simulink model "omav_LBF_hover"  (R2020a)
settings: Solver=VariableStepAuto  StartTime=0.0  StopTime=20  RelTol=1e-3
undefined symbols (not defined in the file): params
libraries: simulink x12, vrlib x1
settings Model: Creator=daniel  LastModifiedBy=daniel

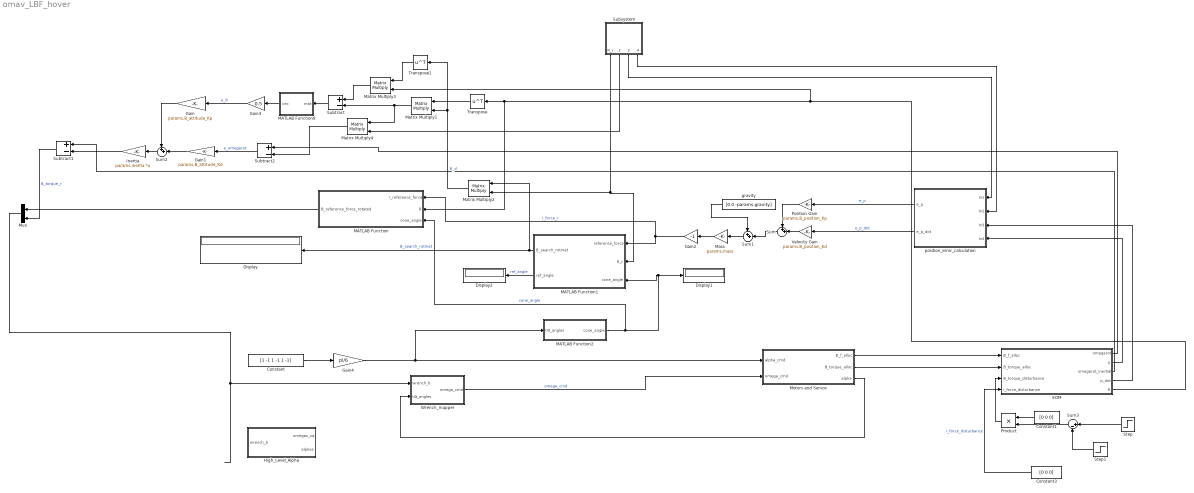
== system omav_LBF_hover ==
  Constant : Constant  Value=[1 -1 1 -1 1 -1]
  Constant1 : Constant  Value=[0 0 0]
  Constant3 : Constant  Value=[0 0 0]
  Display : Display
  Display1 : Display
  Display2 : Display
  EOM : Subsystem
  Gain : Gain  Gain=params.B_attitude_Kp
  Gain1 : Gain  Gain=params.B_attitude_Kd
  Gain2 : Gain  Gain=-1
  Gain3 : Gain  Gain=0.5
  Gain4 : Gain  Gain=pi/6
  High_Level_Alpha : Subsystem
  Inertia : Gain  Gain=params.inertia  Multiplication=Matrix(K*u) (u vector)
  MATLAB Function : MATLAB Function  TreatAsAtomicUnit=on
  MATLAB Function1 : MATLAB Function  TreatAsAtomicUnit=on
  MATLAB Function2 : MATLAB Function  TreatAsAtomicUnit=on
  MATLAB Function8 : MATLAB Function  TreatAsAtomicUnit=on
  Mass : Gain  Gain=params.mass
  Matrix Multiply{1..4} (4 alike) : Product  Multiplication=Matrix(*)
  Motors and Servos : Subsystem
  Mux : Mux  Inputs=2
  Position Gain : Gain  Gain=params.B_position_Kp
  Product : Product
  Step : Step  SampleTime=0
  Step1 : Step  Time=3  SampleTime=0
  Subsystem : Subsystem
  Subtract : Sum  Inputs=+-
  Subtract1 : Sum  Inputs=+-
  Subtract2 : Sum  Inputs=+-
  Sum : Sum  Inputs=++|
  Sum1 : Sum  Inputs=++|
  Sum2 : Sum  Inputs=++|
  Sum3 : Sum  Inputs=|+-
  Transpose : Math  Operator=transpose  SaturateOnIntegerOverflow=on
  Transpose1 : Math  Operator=transpose  SaturateOnIntegerOverflow=on
  Velocity Gain : Gain  Gain=params.B_position_Kd
  Wrench_mapper : Subsystem
  gravity : Constant  Value=[0 0 -params.gravity]
  position_error_calculation : Subsystem
  wires:
  Mux/1 -> Wrench_mapper/1(wrench_b)
  Constant3/1 -> EOM/4(I_force_disturbance)  "I_force_disturbance"
  Motors and Servos/1(B_f_alloc) -> EOM/1(B_f_alloc)
  Motors and Servos/2(B_torque_alloc) -> EOM/2(B_torque_alloc)
  Constant/1 -> Gain4/1
  Motors and Servos/3(alpha) -> Wrench_mapper/2(tilt_angles)
  Wrench_mapper/1(omega_cmd) -> Motors and Servos/2(omega_cmd)  "omega_cmd"
  Velocity Gain/1 -> Sum/2
  Position Gain/1 -> Sum/1
  Sum/1 -> Sum1/2
  gravity/1 -> Sum1/1
  Sum1/1 -> Mass/1
  Gain2/1 -> MATLAB Function1/1(reference_force), MATLAB Function/1(I_reference_force)  "I_force_r"
  MATLAB Function1/1(B_search_rotmat) -> Display/1, Matrix Multiply2/1  "B_search_rotmat"
  Matrix Multiply1/1 -> Subtract/2, Matrix Multiply4/1
  Matrix Multiply4/1 -> Subtract2/2
  EOM/4(p_dot) -> position_error_calculation/3(In3)
  Matrix Multiply3/1 -> Subtract/1
  EOM/5(R) -> Matrix Multiply3/2, MATLAB Function/2(R), Transpose/1
  Transpose1/1 -> Matrix Multiply3/1
  MATLAB Function8/1(vec) -> Gain3/1
  Subtract2/1 -> Gain1/1  "e_omegarot"
  Subtract/1 -> MATLAB Function8/1(mat)
  Transpose/1 -> Matrix Multiply1/1
  EOM/1(omegarot) -> Subtract2/1
  Gain3/1 -> Gain/1  "e_R"
  EOM/2(p) -> position_error_calculation/4(In4)
  position_error_calculation/1(e_p) -> Position Gain/1  "e_p"
  position_error_calculation/2(e_p_dot) -> Velocity Gain/1  "e_p_dot"
  Matrix Multiply2/1 -> Matrix Multiply1/2, Transpose1/1  "R_d"
  Subsystem/2(omega_dot_r) -> Matrix Multiply4/2
  Subsystem/3(Out3) -> position_error_calculation/1(In1)
  Subsystem/4(p_r1) -> position_error_calculation/2(In2)
  Subsystem/1(R_r) -> MATLAB Function1/2(R_r), Matrix Multiply2/2
  EOM/3(omegarot_inertial) -> Subtract1/1
  Gain1/1 -> Sum2/2
  Gain/1 -> Sum2/1
  Sum2/1 -> Inertia/1
  Inertia/1 -> Subtract1/2
  Subtract1/1 -> Mux/2  "B_torque_r"
  Mass/1 -> Gain2/1
  Step/1 -> Sum3/1
  Step1/1 -> Sum3/2
  Sum3/1 -> Product/2
  Constant1/1 -> Product/1
  Product/1 -> EOM/3(B_torque_disturbance)
  Gain4/1 -> MATLAB Function2/1(tilt_angles), Motors and Servos/1(alpha_cmd)
  MATLAB Function2/1(cone_angle) -> MATLAB Function/3(cone_angle), Display1/1, MATLAB Function1/3(cone_angle)  "cone_angle"
  MATLAB Function/1(B_reference_force_rotated) -> Mux/1
  MATLAB Function1/2(ref_angle) -> Display2/1  "ref_angle"

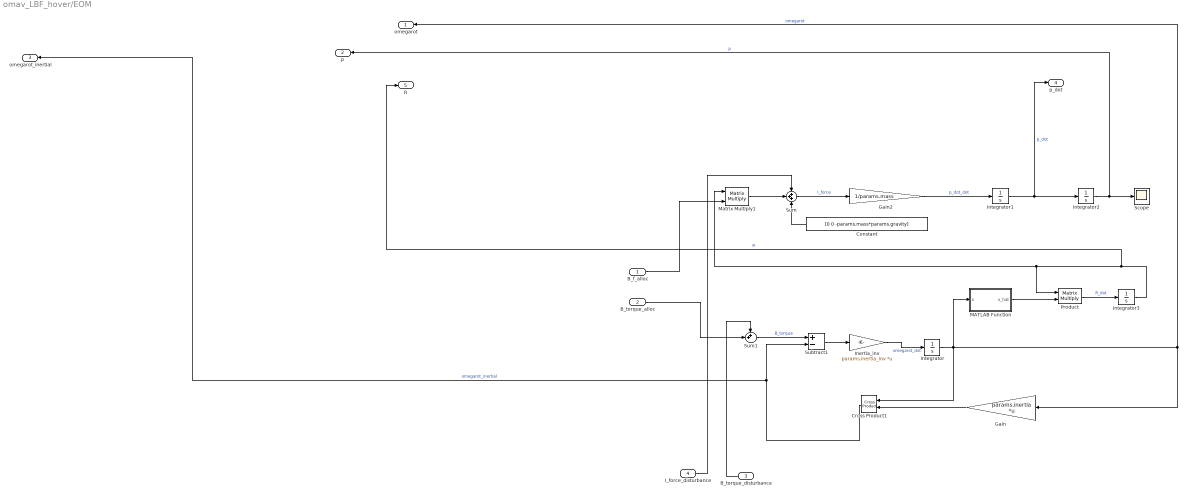
== system omav_LBF_hover/EOM ==
  B_f_alloc : Inport
  B_torque_alloc : Inport  Port=2
  B_torque_disturbance : Inport  Port=3
  I_force_disturbance : Inport  Port=4
  Constant : Constant  Value=[0 0 -params.mass*params.gravity]
  Cross Product1 : vrlib/Utilities/Cross Product
  Gain : Gain  Gain=params.inertia  Multiplication=Matrix(K*u) (u vector)
  Gain2 : Gain  Gain=1/params.mass
  Inertia_inv : Gain  Gain=params.inertia_inv  Multiplication=Matrix(K*u) (u vector)
  Integrator : Integrator
  Integrator1 : Integrator
  Integrator2 : Integrator
  Integrator3 : Integrator  InitialCondition=[1 0 0;0 1 0;0 0 1]
  MATLAB Function : MATLAB Function  TreatAsAtomicUnit=on
  Matrix Multiply1 : Product  Multiplication=Matrix(*)
  Product : Product  Multiplication=Matrix(*)  OutMin=0
  Scope : Scope
  Subtract1 : Sum  Inputs=+-
  Sum : Sum  Inputs=+++
  Sum1 : Sum  Inputs=++|
  omegarot : Outport
  p : Outport  Port=2
  omegarot_inertial : Outport  Port=3
  p_dot : Outport  Port=4
  R : Outport  Port=5
  wires:
  MATLAB Function/1(x_hat) -> Product/2
  Inertia_inv/1 -> Integrator/1  "omegarot_dot"
  Matrix Multiply1/1 -> Sum/2
  Sum1/1 -> Subtract1/1  "B_torque"
  Sum/1 -> Gain2/1  "I_force"
  B_torque_disturbance/1 -> Sum1/1
  Constant/1 -> Sum/3
  Integrator3/1 -> R/1, Product/1, Matrix Multiply1/1  "R"
  Integrator2/1 -> p/1, Scope/1  "p"
  Gain/1 -> Cross Product1/2
  Product/1 -> Integrator3/1  "R_dot"
  Subtract1/1 -> Inertia_inv/1
  Gain2/1 -> Integrator1/1  "p_dot_dot"
  B_f_alloc/1 -> Matrix Multiply1/2
  Cross Product1/1 -> omegarot_inertial/1, Subtract1/2  "omegarot_inertial"
  B_torque_alloc/1 -> Sum1/2
  Integrator/1 -> omegarot/1, Gain/1, MATLAB Function/1(x), Cross Product1/1  "omegarot"
  I_force_disturbance/1 -> Sum/1
  Integrator1/1 -> p_dot/1, Integrator2/1  "p_dot"

== system omav_LBF_hover/High_Level_Alpha ==
  wrench_b : Inport
  MATLAB Function3 : MATLAB Function  TreatAsAtomicUnit=on
  MATLAB Function4 : MATLAB Function  TreatAsAtomicUnit=on
  MATLAB Function5 : MATLAB Function  TreatAsAtomicUnit=on
  omegas_sq : Outport
  alphas : Outport  Port=2
  wires:
  MATLAB Function5/1(X) -> MATLAB Function4/1(X)
  wrench_b/1 -> MATLAB Function5/2(wrench_b)
  MATLAB Function4/2(omegas_sq) -> omegas_sq/1
  MATLAB Function4/1(alphas) -> alphas/1
  MATLAB Function3/1(A) -> MATLAB Function5/1(A)

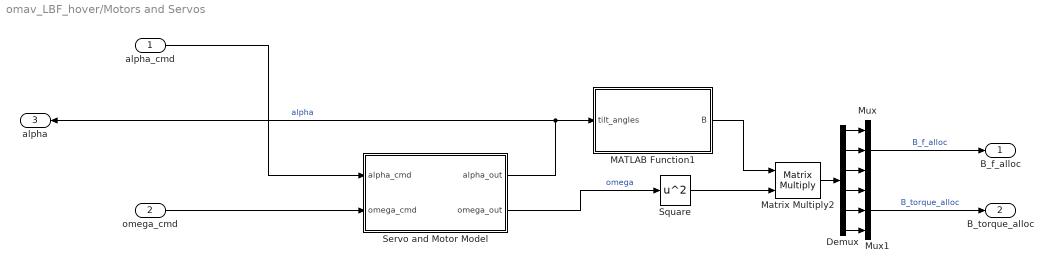
== system omav_LBF_hover/Motors and Servos ==
  alpha_cmd : Inport
  omega_cmd : Inport  Port=2
  Demux : Demux  Outputs=6
  MATLAB Function1 : MATLAB Function  TreatAsAtomicUnit=on
  Matrix Multiply2 : Product  Multiplication=Matrix(*)
  Mux : Mux  Inputs=3
  Mux1 : Mux  Inputs=3
  Servo and Motor Model : Subsystem
  Square : Math  Operator=square  SaturateOnIntegerOverflow=on
  B_f_alloc : Outport
  B_torque_alloc : Outport  Port=2
  alpha : Outport  Port=3
  wires:
  Demux/1 -> Mux/1
  MATLAB Function1/1(B) -> Matrix Multiply2/1
  Demux/4 -> Mux1/1
  Servo and Motor Model/2(omega_out) -> Square/1  "omega"
  Demux/5 -> Mux1/2
  Matrix Multiply2/1 -> Demux/1
  Servo and Motor Model/1(alpha_out) -> alpha/1, MATLAB Function1/1(tilt_angles)  "alpha"
  alpha_cmd/1 -> Servo and Motor Model/1(alpha_cmd)
  Demux/6 -> Mux1/3
  Demux/2 -> Mux/2
  Square/1 -> Matrix Multiply2/2
  omega_cmd/1 -> Servo and Motor Model/2(omega_cmd)
  Mux/1 -> B_f_alloc/1  "B_f_alloc"
  Demux/3 -> Mux/3
  Mux1/1 -> B_torque_alloc/1  "B_torque_alloc"

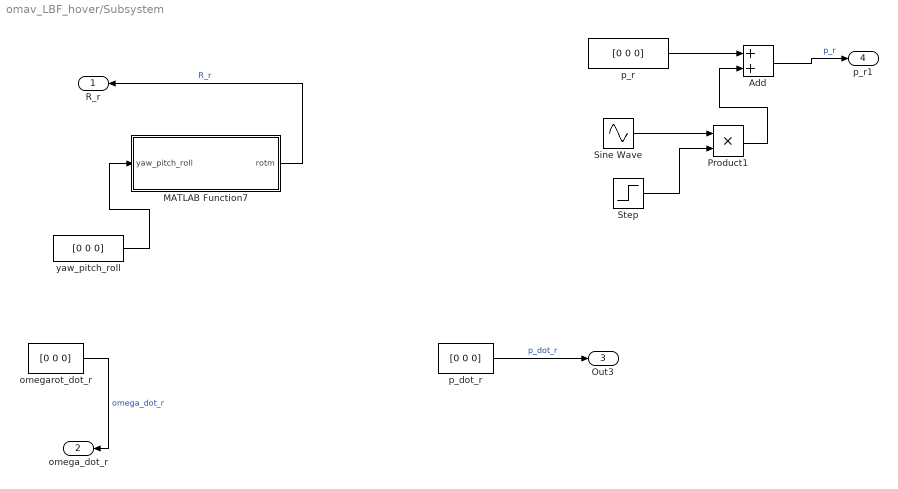
== system omav_LBF_hover/Subsystem ==
  Add : Sum
  MATLAB Function7 : MATLAB Function  TreatAsAtomicUnit=on
  Product1 : Product
  Sine Wave : Sin  Amplitude=[1 0 0]  Frequency=2  SampleTime=0
  Step : Step  Time=3  SampleTime=0
  omegarot_dot_r : Constant  Value=[0 0 0]
  p_dot_r : Constant  Value=[0 0 0]
  p_r : Constant  Value=[0 0 0]
  yaw_pitch_roll : Constant  Value=[0 0 0]
  R_r : Outport
  omega_dot_r : Outport  Port=2
  Out3 : Outport  Port=3
  p_r1 : Outport  Port=4
  wires:
  Step/1 -> Product1/2
  omegarot_dot_r/1 -> omega_dot_r/1  "omega_dot_r"
  Add/1 -> p_r1/1  "p_r"
  yaw_pitch_roll/1 -> MATLAB Function7/1(yaw_pitch_roll)
  MATLAB Function7/1(rotm) -> R_r/1  "R_r"
  Product1/1 -> Add/2
  p_dot_r/1 -> Out3/1  "p_dot_r"
  Sine Wave/1 -> Product1/1
  p_r/1 -> Add/1

== system omav_LBF_hover/Wrench_mapper ==
  wrench_b : Inport
  tilt_angles : Inport  Port=2
  MATLAB Function2 : MATLAB Function  TreatAsAtomicUnit=on
  MATLAB Function6 : MATLAB Function  TreatAsAtomicUnit=on
  Sqrt : Sqrt  SaturateOnIntegerOverflow=on
  omega_cmd : Outport
  wires:
  wrench_b/1 -> MATLAB Function2/2(wrench_b)
  Sqrt/1 -> omega_cmd/1  "omega_cmd"
  MATLAB Function2/1(omega_sq) -> Sqrt/1
  MATLAB Function6/1(B) -> MATLAB Function2/1(B)
  tilt_angles/1 -> MATLAB Function6/1(tilt_angles)

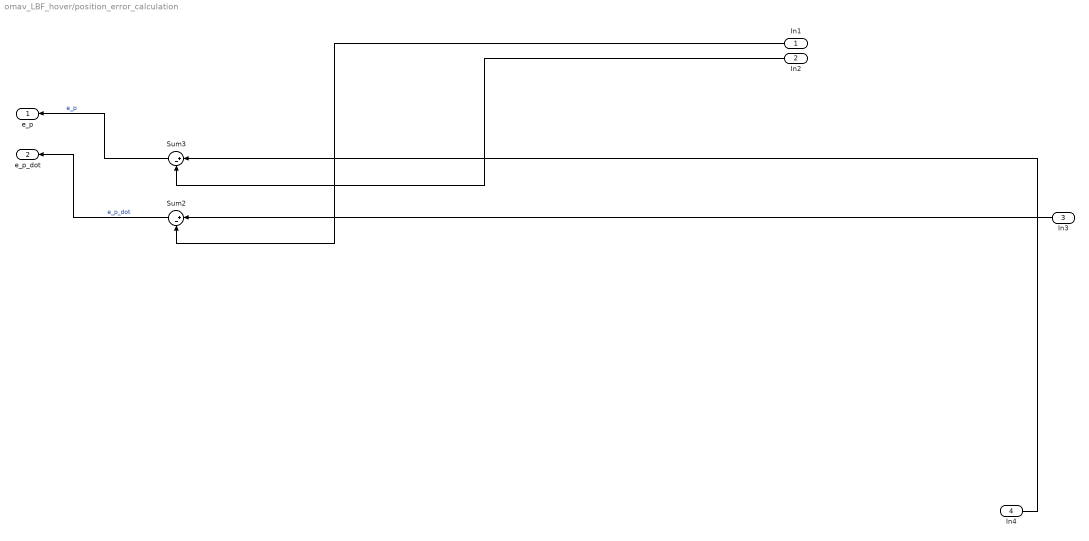
== system omav_LBF_hover/position_error_calculation ==
  In1 : Inport
  In2 : Inport  Port=2
  In3 : Inport  Port=3
  In4 : Inport  Port=4
  Sum2 : Sum  Inputs=|+-
  Sum3 : Sum  Inputs=|+-
  e_p : Outport
  e_p_dot : Outport  Port=2
  wires:
  Sum2/1 -> e_p_dot/1  "e_p_dot"
  In3/1 -> Sum2/1
  In4/1 -> Sum3/1
  In1/1 -> Sum2/2
  Sum3/1 -> e_p/1  "e_p"
  In2/1 -> Sum3/2

== system omav_LBF_hover/Motors and Servos/Servo and Motor Model ==
  alpha_cmd : Inport
  omega_cmd : Inport  Port=2
  all_rotors_subsystem1 : Subsystem
      mask Display: image('images/brushless.JPG'); % Use "Edit Image" on toolstrip to change.
  all_servos_subsystem1 : Subsystem
      mask Display: image('images/servo.jpg'); % Use "Edit Image" on toolstrip to change.
  alpha_out : Outport
  omega_out : Outport  Port=2
  wires:
  alpha_cmd/1 -> all_servos_subsystem1/1(alphas_cmd)  "alpha_cmd"
  all_rotors_subsystem1/1(omegas_out) -> omega_out/1  "omega_out"
  all_servos_subsystem1/1(alphas_out) -> alpha_out/1  "alpha_out"
  omega_cmd/1 -> all_rotors_subsystem1/1(omegas_cmd)  "omega_cmd"

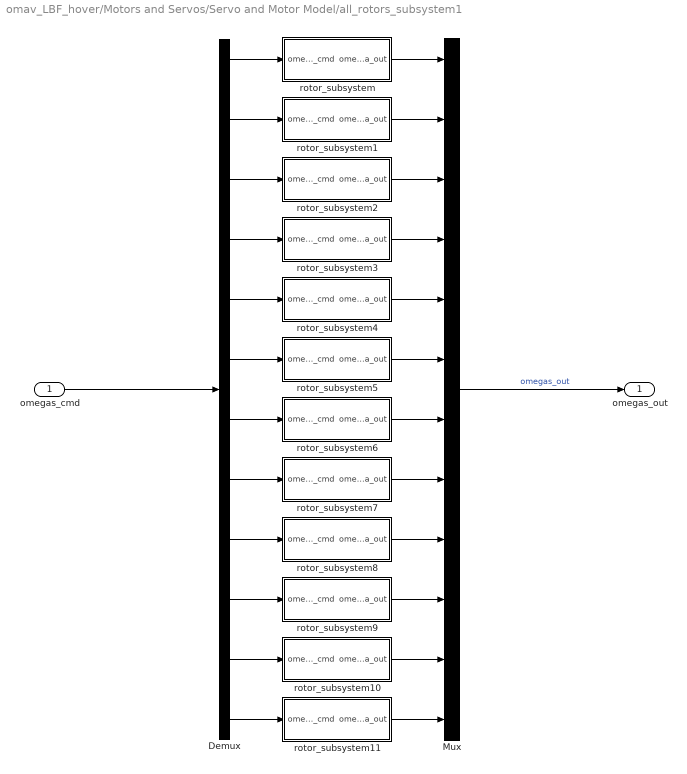
== system omav_LBF_hover/Motors and Servos/Servo and Motor Model/all_rotors_subsystem1 ==
  omegas_cmd : Inport
  Demux : Demux  Outputs=12
  Mux : Mux  Inputs=12
  rotor_subsystem : Subsystem
  rotor_subsystem1 : Subsystem
  rotor_subsystem10 : Subsystem
  rotor_subsystem11 : Subsystem
  rotor_subsystem2 : Subsystem
  rotor_subsystem3 : Subsystem
  rotor_subsystem4 : Subsystem
  rotor_subsystem5 : Subsystem
  rotor_subsystem6 : Subsystem
  rotor_subsystem7 : Subsystem
  rotor_subsystem8 : Subsystem
  rotor_subsystem9 : Subsystem
  omegas_out : Outport
  wires:
  Demux/3 -> rotor_subsystem2/1(omega_cmd)
  rotor_subsystem10/1(omega_out) -> Mux/11
  rotor_subsystem7/1(omega_out) -> Mux/8
  rotor_subsystem2/1(omega_out) -> Mux/3
  rotor_subsystem1/1(omega_out) -> Mux/2
  Demux/2 -> rotor_subsystem1/1(omega_cmd)
  rotor_subsystem5/1(omega_out) -> Mux/6
  rotor_subsystem4/1(omega_out) -> Mux/5
  Demux/4 -> rotor_subsystem3/1(omega_cmd)
  rotor_subsystem6/1(omega_out) -> Mux/7
  Demux/8 -> rotor_subsystem7/1(omega_cmd)
  rotor_subsystem/1(omega_out) -> Mux/1
  rotor_subsystem3/1(omega_out) -> Mux/4
  rotor_subsystem11/1(omega_out) -> Mux/12
  rotor_subsystem8/1(omega_out) -> Mux/9
  Demux/11 -> rotor_subsystem10/1(omega_cmd)
  rotor_subsystem9/1(omega_out) -> Mux/10
  Demux/1 -> rotor_subsystem/1(omega_cmd)
  omegas_cmd/1 -> Demux/1
  Mux/1 -> omegas_out/1  "omegas_out"
  Demux/12 -> rotor_subsystem11/1(omega_cmd)
  Demux/10 -> rotor_subsystem9/1(omega_cmd)
  Demux/9 -> rotor_subsystem8/1(omega_cmd)
  Demux/7 -> rotor_subsystem6/1(omega_cmd)
  Demux/6 -> rotor_subsystem5/1(omega_cmd)
  Demux/5 -> rotor_subsystem4/1(omega_cmd)

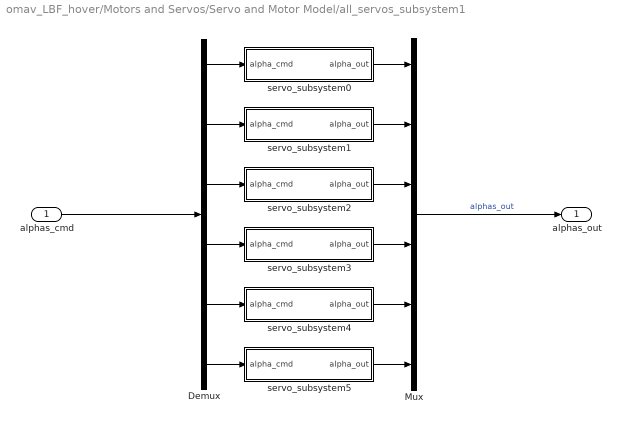
== system omav_LBF_hover/Motors and Servos/Servo and Motor Model/all_servos_subsystem1 ==
  alphas_cmd : Inport
  Demux : Demux  Outputs=6
  Mux : Mux  Inputs=6
  servo_subsystem0 : Subsystem
  servo_subsystem1 : Subsystem
  servo_subsystem2 : Subsystem
  servo_subsystem3 : Subsystem
  servo_subsystem4 : Subsystem
  servo_subsystem5 : Subsystem
  alphas_out : Outport
  wires:
  alphas_cmd/1 -> Demux/1
  Demux/2 -> servo_subsystem1/1(alpha_cmd)
  servo_subsystem3/1(alpha_out) -> Mux/4
  servo_subsystem1/1(alpha_out) -> Mux/2
  Demux/4 -> servo_subsystem3/1(alpha_cmd)
  servo_subsystem4/1(alpha_out) -> Mux/5
  Demux/5 -> servo_subsystem4/1(alpha_cmd)
  Demux/1 -> servo_subsystem0/1(alpha_cmd)
  servo_subsystem2/1(alpha_out) -> Mux/3
  servo_subsystem5/1(alpha_out) -> Mux/6
  Demux/6 -> servo_subsystem5/1(alpha_cmd)
  Demux/3 -> servo_subsystem2/1(alpha_cmd)
  Mux/1 -> alphas_out/1  "alphas_out"
  servo_subsystem0/1(alpha_out) -> Mux/1

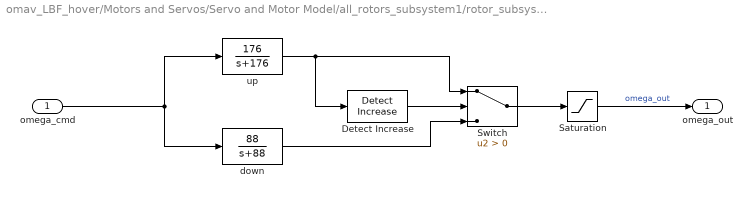
== system omav_LBF_hover/Motors and Servos/Servo and Motor Model/all_rotors_subsystem1/rotor_subsystem ==
  omega_cmd : Inport
  Detect Increase : simulink/Logic and Bit Operations/Detect Increase  vinit=0.0  OutDataTypeStr=boolean
  Saturation : Saturate  UpperLimit=params.rotor_max  LowerLimit=0
  Switch : Switch  Criteria=u2 > Threshold
  down : TransferFcn  Numerator=[88]  Denominator=[1 88]
  up : TransferFcn  Numerator=[176]  Denominator=[1 176]
  omega_out : Outport
  wires:
  down/1 -> Switch/3
  up/1 -> Detect Increase/1, Switch/1
  omega_cmd/1 -> up/1, down/1
  Switch/1 -> Saturation/1
  Detect Increase/1 -> Switch/2
  Saturation/1 -> omega_out/1  "omega_out"

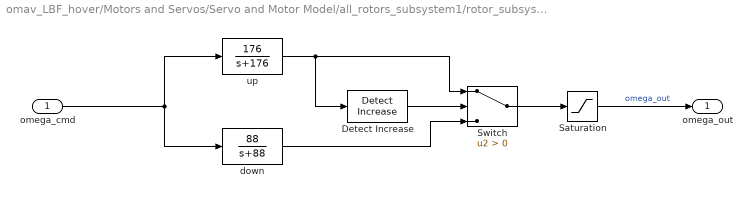
== system omav_LBF_hover/Motors and Servos/Servo and Motor Model/all_rotors_subsystem1/rotor_subsystem1 ==
  omega_cmd : Inport
  Detect Increase : simulink/Logic and Bit Operations/Detect Increase  vinit=0.0  OutDataTypeStr=boolean
  Saturation : Saturate  UpperLimit=params.rotor_max  LowerLimit=0
  Switch : Switch  Criteria=u2 > Threshold
  down : TransferFcn  Numerator=[88]  Denominator=[1 88]
  up : TransferFcn  Numerator=[176]  Denominator=[1 176]
  omega_out : Outport
  wires:
  Saturation/1 -> omega_out/1  "omega_out"
  Detect Increase/1 -> Switch/2
  Switch/1 -> Saturation/1
  omega_cmd/1 -> down/1, up/1
  up/1 -> Switch/1, Detect Increase/1
  down/1 -> Switch/3

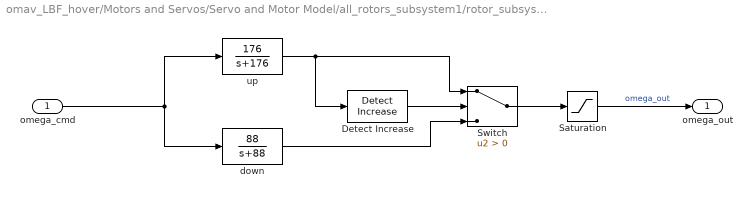
== system omav_LBF_hover/Motors and Servos/Servo and Motor Model/all_rotors_subsystem1/rotor_subsystem10 ==
  omega_cmd : Inport
  Detect Increase : simulink/Logic and Bit Operations/Detect Increase  vinit=0.0  OutDataTypeStr=boolean
  Saturation : Saturate  UpperLimit=params.rotor_max  LowerLimit=0
  Switch : Switch  Criteria=u2 > Threshold
  down : TransferFcn  Numerator=[88]  Denominator=[1 88]
  up : TransferFcn  Numerator=[176]  Denominator=[1 176]
  omega_out : Outport
  wires:
  down/1 -> Switch/3
  up/1 -> Detect Increase/1, Switch/1
  omega_cmd/1 -> up/1, down/1
  Switch/1 -> Saturation/1
  Detect Increase/1 -> Switch/2
  Saturation/1 -> omega_out/1  "omega_out"

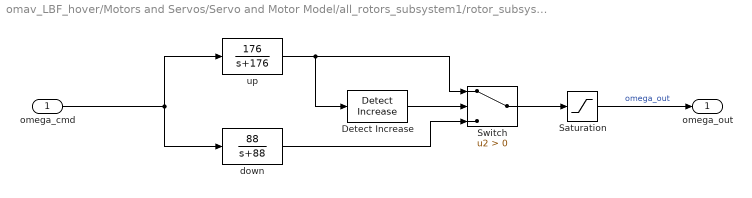
== system omav_LBF_hover/Motors and Servos/Servo and Motor Model/all_rotors_subsystem1/rotor_subsystem11 ==
  omega_cmd : Inport
  Detect Increase : simulink/Logic and Bit Operations/Detect Increase  vinit=0.0  OutDataTypeStr=boolean
  Saturation : Saturate  UpperLimit=params.rotor_max  LowerLimit=0
  Switch : Switch  Criteria=u2 > Threshold
  down : TransferFcn  Numerator=[88]  Denominator=[1 88]
  up : TransferFcn  Numerator=[176]  Denominator=[1 176]
  omega_out : Outport
  wires:
  Saturation/1 -> omega_out/1  "omega_out"
  Detect Increase/1 -> Switch/2
  Switch/1 -> Saturation/1
  omega_cmd/1 -> down/1, up/1
  up/1 -> Switch/1, Detect Increase/1
  down/1 -> Switch/3

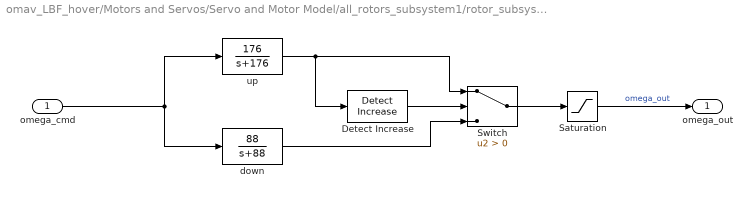
== system omav_LBF_hover/Motors and Servos/Servo and Motor Model/all_rotors_subsystem1/rotor_subsystem2 ==
  omega_cmd : Inport
  Detect Increase : simulink/Logic and Bit Operations/Detect Increase  vinit=0.0  OutDataTypeStr=boolean
  Saturation : Saturate  UpperLimit=params.rotor_max  LowerLimit=0
  Switch : Switch  Criteria=u2 > Threshold
  down : TransferFcn  Numerator=[88]  Denominator=[1 88]
  up : TransferFcn  Numerator=[176]  Denominator=[1 176]
  omega_out : Outport
  wires:
  down/1 -> Switch/3
  up/1 -> Detect Increase/1, Switch/1
  omega_cmd/1 -> up/1, down/1
  Switch/1 -> Saturation/1
  Detect Increase/1 -> Switch/2
  Saturation/1 -> omega_out/1  "omega_out"

== system omav_LBF_hover/Motors and Servos/Servo and Motor Model/all_rotors_subsystem1/rotor_subsystem3 ==
  omega_cmd : Inport
  Detect Increase : simulink/Logic and Bit Operations/Detect Increase  vinit=0.0  OutDataTypeStr=boolean
  Saturation : Saturate  UpperLimit=params.rotor_max  LowerLimit=0
  Switch : Switch  Criteria=u2 > Threshold
  down : TransferFcn  Numerator=[88]  Denominator=[1 88]
  up : TransferFcn  Numerator=[176]  Denominator=[1 176]
  omega_out : Outport
  wires:
  Saturation/1 -> omega_out/1  "omega_out"
  Detect Increase/1 -> Switch/2
  Switch/1 -> Saturation/1
  omega_cmd/1 -> down/1, up/1
  up/1 -> Switch/1, Detect Increase/1
  down/1 -> Switch/3

== system omav_LBF_hover/Motors and Servos/Servo and Motor Model/all_rotors_subsystem1/rotor_subsystem4 ==
  omega_cmd : Inport
  Detect Increase : simulink/Logic and Bit Operations/Detect Increase  vinit=0.0  OutDataTypeStr=boolean
  Saturation : Saturate  UpperLimit=params.rotor_max  LowerLimit=0
  Switch : Switch  Criteria=u2 > Threshold
  down : TransferFcn  Numerator=[88]  Denominator=[1 88]
  up : TransferFcn  Numerator=[176]  Denominator=[1 176]
  omega_out : Outport
  wires:
  down/1 -> Switch/3
  up/1 -> Detect Increase/1, Switch/1
  omega_cmd/1 -> up/1, down/1
  Switch/1 -> Saturation/1
  Detect Increase/1 -> Switch/2
  Saturation/1 -> omega_out/1  "omega_out"

== system omav_LBF_hover/Motors and Servos/Servo and Motor Model/all_rotors_subsystem1/rotor_subsystem5 ==
  omega_cmd : Inport
  Detect Increase : simulink/Logic and Bit Operations/Detect Increase  vinit=0.0  OutDataTypeStr=boolean
  Saturation : Saturate  UpperLimit=params.rotor_max  LowerLimit=0
  Switch : Switch  Criteria=u2 > Threshold
  down : TransferFcn  Numerator=[88]  Denominator=[1 88]
  up : TransferFcn  Numerator=[176]  Denominator=[1 176]
  omega_out : Outport
  wires:
  Saturation/1 -> omega_out/1  "omega_out"
  Detect Increase/1 -> Switch/2
  Switch/1 -> Saturation/1
  omega_cmd/1 -> down/1, up/1
  up/1 -> Switch/1, Detect Increase/1
  down/1 -> Switch/3

== system omav_LBF_hover/Motors and Servos/Servo and Motor Model/all_rotors_subsystem1/rotor_subsystem6 ==
  omega_cmd : Inport
  Detect Increase : simulink/Logic and Bit Operations/Detect Increase  vinit=0.0  OutDataTypeStr=boolean
  Saturation : Saturate  UpperLimit=params.rotor_max  LowerLimit=0
  Switch : Switch  Criteria=u2 > Threshold
  down : TransferFcn  Numerator=[88]  Denominator=[1 88]
  up : TransferFcn  Numerator=[176]  Denominator=[1 176]
  omega_out : Outport
  wires:
  down/1 -> Switch/3
  up/1 -> Detect Increase/1, Switch/1
  omega_cmd/1 -> up/1, down/1
  Switch/1 -> Saturation/1
  Detect Increase/1 -> Switch/2
  Saturation/1 -> omega_out/1  "omega_out"

== system omav_LBF_hover/Motors and Servos/Servo and Motor Model/all_rotors_subsystem1/rotor_subsystem7 ==
  omega_cmd : Inport
  Detect Increase : simulink/Logic and Bit Operations/Detect Increase  vinit=0.0  OutDataTypeStr=boolean
  Saturation : Saturate  UpperLimit=params.rotor_max  LowerLimit=0
  Switch : Switch  Criteria=u2 > Threshold
  down : TransferFcn  Numerator=[88]  Denominator=[1 88]
  up : TransferFcn  Numerator=[176]  Denominator=[1 176]
  omega_out : Outport
  wires:
  Saturation/1 -> omega_out/1  "omega_out"
  Detect Increase/1 -> Switch/2
  Switch/1 -> Saturation/1
  omega_cmd/1 -> down/1, up/1
  up/1 -> Switch/1, Detect Increase/1
  down/1 -> Switch/3

== system omav_LBF_hover/Motors and Servos/Servo and Motor Model/all_rotors_subsystem1/rotor_subsystem8 ==
  omega_cmd : Inport
  Detect Increase : simulink/Logic and Bit Operations/Detect Increase  vinit=0.0  OutDataTypeStr=boolean
  Saturation : Saturate  UpperLimit=params.rotor_max  LowerLimit=0
  Switch : Switch  Criteria=u2 > Threshold
  down : TransferFcn  Numerator=[88]  Denominator=[1 88]
  up : TransferFcn  Numerator=[176]  Denominator=[1 176]
  omega_out : Outport
  wires:
  down/1 -> Switch/3
  up/1 -> Detect Increase/1, Switch/1
  omega_cmd/1 -> up/1, down/1
  Switch/1 -> Saturation/1
  Detect Increase/1 -> Switch/2
  Saturation/1 -> omega_out/1  "omega_out"

== system omav_LBF_hover/Motors and Servos/Servo and Motor Model/all_rotors_subsystem1/rotor_subsystem9 ==
  omega_cmd : Inport
  Detect Increase : simulink/Logic and Bit Operations/Detect Increase  vinit=0.0  OutDataTypeStr=boolean
  Saturation : Saturate  UpperLimit=params.rotor_max  LowerLimit=0
  Switch : Switch  Criteria=u2 > Threshold
  down : TransferFcn  Numerator=[88]  Denominator=[1 88]
  up : TransferFcn  Numerator=[176]  Denominator=[1 176]
  omega_out : Outport
  wires:
  Saturation/1 -> omega_out/1  "omega_out"
  Detect Increase/1 -> Switch/2
  Switch/1 -> Saturation/1
  omega_cmd/1 -> down/1, up/1
  up/1 -> Switch/1, Detect Increase/1
  down/1 -> Switch/3

== system omav_LBF_hover/Motors and Servos/Servo and Motor Model/all_servos_subsystem1/servo_subsystem0 ==
  alpha_cmd : Inport
  Servo Transfer Function : TransferFcn  Numerator=[256]  Denominator=[1 22.4 256]
  alpha_out : Outport
  wires:
  alpha_cmd/1 -> Servo Transfer Function/1
  Servo Transfer Function/1 -> alpha_out/1  "alpha_out"

== system omav_LBF_hover/Motors and Servos/Servo and Motor Model/all_servos_subsystem1/servo_subsystem1 ==
  alpha_cmd : Inport
  Servo Transfer Function : TransferFcn  Numerator=[256]  Denominator=[1 22.4 256]
  alpha_out : Outport
  wires:
  Servo Transfer Function/1 -> alpha_out/1  "alpha_out"
  alpha_cmd/1 -> Servo Transfer Function/1

== system omav_LBF_hover/Motors and Servos/Servo and Motor Model/all_servos_subsystem1/servo_subsystem2 ==
  alpha_cmd : Inport
  Servo Transfer Function : TransferFcn  Numerator=[256]  Denominator=[1 22.4 256]
  alpha_out : Outport
  wires:
  alpha_cmd/1 -> Servo Transfer Function/1
  Servo Transfer Function/1 -> alpha_out/1  "alpha_out"

== system omav_LBF_hover/Motors and Servos/Servo and Motor Model/all_servos_subsystem1/servo_subsystem3 ==
  alpha_cmd : Inport
  Servo Transfer Function : TransferFcn  Numerator=[256]  Denominator=[1 22.4 256]
  alpha_out : Outport
  wires:
  Servo Transfer Function/1 -> alpha_out/1  "alpha_out"
  alpha_cmd/1 -> Servo Transfer Function/1

== system omav_LBF_hover/Motors and Servos/Servo and Motor Model/all_servos_subsystem1/servo_subsystem4 ==
  alpha_cmd : Inport
  Servo Transfer Function : TransferFcn  Numerator=[256]  Denominator=[1 22.4 256]
  alpha_out : Outport
  wires:
  alpha_cmd/1 -> Servo Transfer Function/1
  Servo Transfer Function/1 -> alpha_out/1  "alpha_out"

== system omav_LBF_hover/Motors and Servos/Servo and Motor Model/all_servos_subsystem1/servo_subsystem5 ==
  alpha_cmd : Inport
  Servo Transfer Function : TransferFcn  Numerator=[256]  Denominator=[1 22.4 256]
  alpha_out : Outport
  wires:
  Servo Transfer Function/1 -> alpha_out/1  "alpha_out"
  alpha_cmd/1 -> Servo Transfer Function/1

== matlab function omav_LBF_hover/Motors and Servos/MATLAB Function1 ==
  data: tilt_angles input; B output
function B = get_B(tilt_angles)
%tilt_angles [6x1]
%[F, tau] = B * [omega²]

params = parameters();

rotor_force_constant = params.rotor_force_constant;
rotor_moment_constant = params.rotor_moment_constant;
arm_length = params.arm_length;

arm_angles = params.arm_angles;
spin = params.spin;

B = zeros(6,12);


j = 0;

%repeat every tilt angle
rep_tilt_angles = repelem(tilt_angles,2);
%iterating through every rotor
%refactored to z-upwards
for i = 1:12
  
    tilt_angle = rep_tilt_angles(i);
    
    B(1,i) = sin(arm_angles(i))*sin(tilt_angle);
    B(2,i) = -cos(arm_angles(i))*sin(tilt_angle);
    B(3,i) = cos(tilt_angle);
    B(4,i) = -(rotor_moment_constant*spin(i)*sin(tilt_angle) - cos(tilt_angle)*arm_length)*sin(arm_angles(i));
    B(5,i) =  (rotor_moment_constant*spin(i)*sin(tilt_angle) - cos(tilt_angle)*arm_length)*cos(arm_angles(i));
    B(6,i) = -(rotor_moment_constant*spin(i)*cos(tilt_angle) + sin(tilt_angle)*arm_length);
end

B = B*rotor_force_constant;

== matlab function omav_LBF_hover/EOM/MATLAB Function ==
  data: x input; x_hat output
function x_hat = hat_map(x)
x_hat = [0 -x(3) x(2); x(3) 0 -x(1); -x(2) x(1) 0];

== matlab function omav_LBF_hover/Wrench_mapper/MATLAB Function2 ==
  data: B input; omega_sq output; wrench_b input
function omega_sq = get_omegasq(B,wrench_b)
%GET_OMEGASQ Summary of this function goes here
%   Detailed explanation goes here

params = parameters();
omega_sq = pinv(B)*wrench_b;

for i = 1:12
    if omega_sq(i) < 0
        omega_sq(i) = 0;
    end
    
    if omega_sq(i) > (params.rotor_max)^2
        omega_sq(i) = (params.rotor_max)^2;
    end
end

end

== matlab function omav_LBF_hover/High_Level_Alpha/MATLAB Function3 ==
  data: A output
function A = get_A()
%[F, tau] = A * [sin(alpha)*omega², cos(alpha)*omega²]

params = parameters();

rotor_force_constant = params.rotor_force_constant;
rotor_moment_constant = params.rotor_moment_constant;
arm_length = params.arm_length;

arm_angles = params.arm_angles;
spin = params.spin;

%implementing pre-calculated matrix
%zero entries are commented out
A = zeros(6,24);

%iterating through every rotor
%refactored to z-up coordinate system
for i = 1:12
    A(1,2*i-1) = sin(arm_angles(i));
    %A(1,2*i) = 0;
    
    A(2,2*i-1) = -cos(arm_angles(i));
    %A(2,2*i) = 0;
    
    %A(3,2*i-1) = 0;
    A(3,2*i) = 1;
    
    A(4,2*i-1) = -rotor_moment_constant*spin(i)*sin(arm_angles(i));
    A(4,2*i) = sin(arm_angles(i))*arm_length;
    
    A(5,2*i-1) = rotor_moment_constant*spin(i)*cos(arm_angles(i));
    A(5,2*i) = -cos(arm_angles(i))*arm_length;
    
    A(6,2*i-1) = -arm_length;
    A(6,2*i) = -rotor_moment_constant*spin(i);
end

%multiplying with rotor force constant
A = A*rotor_force_constant;

== matlab function omav_LBF_hover/High_Level_Alpha/MATLAB Function4 ==
  data: X input; alphas output; omegas_sq output
function [alphas, omegas_sq] = get_projections(X)
%GET_PROJECTIONS Summary of this function goes here
%   Detailed explanation goes here


%get the angles
alphas = zeros(6,1);
for i = 1:6
    %get to entry which corresponds to arm
    j = 4*i - 3;
    alphas(i) = atan2(X(j)+X(j+2),X(j+1)+X(j+3));
end

omegas_sq = zeros(12,1);
for i = 1:6
    %get to entry which corresponds to arm
    j = 4*i - 3;
    
    omegas_sq(2*i-1) = X(j)*sin(alphas(i)) + X(j+1)*cos(alphas(i));
    omegas_sq(2*i)   = X(j+2)*sin(alphas(i)) + X(j+3)*cos(alphas(i));
end

%set to zero if smaller than zero
for i = 1:12
    if omegas_sq(i) < 0
        omegas_sq(i) = 0;
    end
end

== matlab function omav_LBF_hover/High_Level_Alpha/MATLAB Function5 ==
  data: A input; X output; wrench_b input
function X = get_X(A,wrench_b)
%GET_X Summary of this function goes here
%   Detailed explanation goes here
wrench_b = wrench_b(:);

X = pinv(A)*wrench_b;
end

== matlab function omav_LBF_hover/Wrench_mapper/MATLAB Function6 ==
  data: tilt_angles input; B output
function B = get_B(tilt_angles)
%tilt_angles [6x1]
%[F, tau] = B * [omega²]

params = parameters();

rotor_force_constant = params.rotor_force_constant;
rotor_moment_constant = params.rotor_moment_constant;
arm_length = params.arm_length;

arm_angles = params.arm_angles;
spin = params.spin;

B = zeros(6,12);


j = 0;

%repeat every tilt angle
rep_tilt_angles = repelem(tilt_angles,2);
%iterating through every rotor
%refactored to z-upwards
for i = 1:12
  
    tilt_angle = rep_tilt_angles(i);
    
    B(1,i) = sin(arm_angles(i))*sin(tilt_angle);
    B(2,i) = -cos(arm_angles(i))*sin(tilt_angle);
    B(3,i) = cos(tilt_angle);
    B(4,i) = -(rotor_moment_constant*spin(i)*sin(tilt_angle) - cos(tilt_angle)*arm_length)*sin(arm_angles(i));
    B(5,i) =  (rotor_moment_constant*spin(i)*sin(tilt_angle) - cos(tilt_angle)*arm_length)*cos(arm_angles(i));
    B(6,i) = -(rotor_moment_constant*spin(i)*cos(tilt_angle) + sin(tilt_angle)*arm_length);
end

B = B*rotor_force_constant;

== matlab function omav_LBF_hover/Subsystem/MATLAB Function7 ==
  data: yaw_pitch_roll input; rotm output
function rotm = fcn(yaw_pitch_roll)
yaw_pitch_roll = yaw_pitch_roll(:)';
rotm = eul2rotm(yaw_pitch_roll);

== matlab function omav_LBF_hover/MATLAB Function8 ==
  data: mat input; vec output
function vec = vee_map(mat)

vec = [-mat(2,3); mat(1,3); -mat(1,2)];

== matlab function omav_LBF_hover/MATLAB Function ==
  data: I_reference_force input; B_reference_force_rotated output; R input; cone_angle input
function B_reference_force_rotated = get_reference_force_rotated(I_reference_force, R, cone_angle)

%normalize reference force vector
I_e_ref = I_reference_force / norm(I_reference_force);

%get reference force vector in body frame
B_e_ref = R'*I_e_ref;

%get reference force angle w.r.t body z axis
ref_angle = acos(I_e_ref(3));

%compare it to force cone_angle
if ref_angle < cone_angle
    %reference force lies within the cone
    B_force_rotmat = eye(3);
else
    %get minimum tilt angle change
    delta_angle = ref_angle - cone_angle;
   
    %get direction orth. to e_z and e_ref
    u = cross([0;0;1],B_e_ref);
    
    %rotate about u
    axang = [u;delta_angle]';
    
    B_force_rotmat = axang2rotm(axang);
end

B_reference_force_rotated = B_force_rotmat*R*I_reference_force;

== matlab function omav_LBF_hover/MATLAB Function1 ==
  data: reference_force input; R_r input; B_search_rotmat output; cone_angle input; ref_angle output
function [B_search_rotmat,ref_angle]  = get_search_rotmat(reference_force,R_r, cone_angle)

%normalize reference force vector
I_e_ref = reference_force / norm(reference_force);

%get reference force vector in desired body frame
B_e_ref = R_r'*I_e_ref;

%get reference force angle w.r.t body z axis
ref_angle = acos(I_e_ref(3));

B_search_rotmat = eye(3);

%compare it to force cone_angle
if ref_angle < cone_angle
    %reference force lies within the cone
    B_search_rotmat = eye(3);
else
    %get minimum tilt angle change
    delta_angle = ref_angle - cone_angle;
   
    %get direction orth. to e_z and e_ref
    u = cross([0;0;1],B_e_ref);
    
    %rotate about u
    axang = [u;delta_angle]';
    
    B_search_rotmat = axang2rotm(axang);
end

== matlab function omav_LBF_hover/MATLAB Function2 ==
  data: tilt_angles input; cone_angle output
function cone_angle = get_cone_angle(tilt_angles)

%assert that tilt angles are symmetric
assert(sum(tilt_angles)==0);

%get gain
k = mean(abs(tilt_angles));

%get cone slope
%TODO: write in parameter file
a = 1.7 / k^1.2;

%get cone angle
cone_angle = asin(1/a);
